simulink model "windpmsg11088"  (R2022b)
settings: Solver=VariableStepAuto  StartTime=0.0  StopTime=10  RelTol=1e-3
undefined symbols (not defined in the file or in its folder): sigbuilder_block
libraries: powerlib_extras x2, spsMeanLib x2, spsThreePhaseVIMeasurementLib x1, spsGroundLib x1, spsCurrentMeasurementLib x1, spsPermanentMagnetSynchronousMachineLib x1, spsThreePhaseSeriesRLCBranchLib x1, spsVoltageMeasurementLib x1, spspowerguiLib x1
settings Model: Creator=CC  LastModifiedBy=admin
settings SolverCC: AlgebraicLoopSolver=TrustRegion
settings DataIOCC: ReturnWorkspaceOutputs=off
settings DebuggingCC: UnconnectedInputMsg=warning  UnconnectedOutputMsg=warning  UnconnectedLineMsg=warning  SFMachineParentedDataDiag=warning  ArithmeticOperatorsInVariantConditions=warning
settings ModelReferenceCC: EnableRefExpFcnMdlSchedulingChecks=on
settings SFSimCC: SimUseLocalCustomCode=off  CustomCodeUndefinedFunction=UseInterfaceOnly
settings RTWCC: RTWUseLocalCustomCode=off

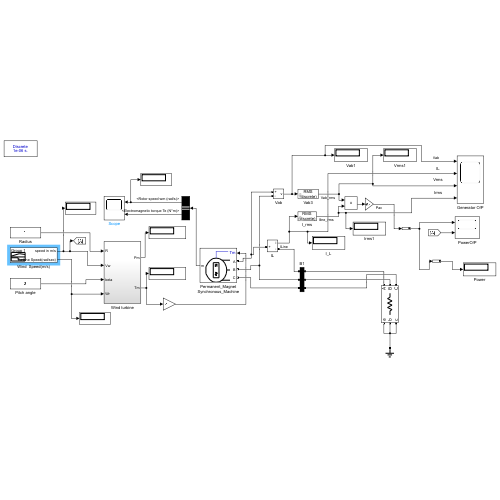
[thumbnail: Simulink's stored preview of the top-level diagram]
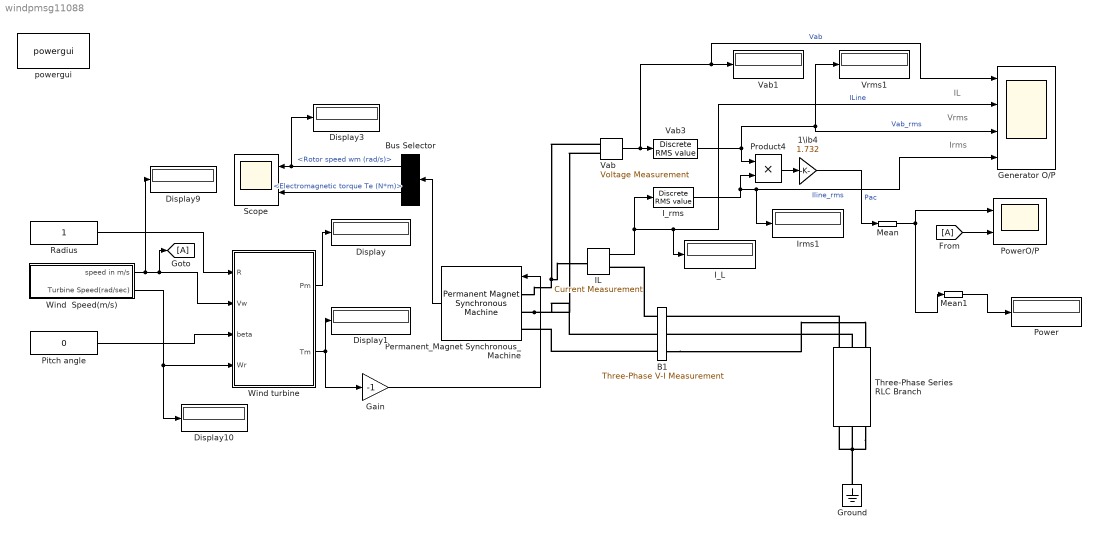
== system windpmsg11088 ==
  note: Irms
  note: Vrms
  note: IL
  1\ib4 : Gain  Gain=1.732  SaturateOnIntegerOverflow=on  OutDataTypeStr=Inherit: Same as input  ParamDataTypeStr=Inherit: Same as input
  B1 : spsThreePhaseVIMeasurementLib/Three-Phase V-I Measurement  VoltageMeasurement=phase-to-ground  SetLabelV=on  LabelV=Vabc_B1  Vpu=off  VpuLL=off  CurrentMeasurement=yes  SetLabelI=on  LabelI=Iabc_B1  Ipu=off  Pbase=100e6  Vbase=500e3  OutputType=Magnitude  PhasorSimulation=off  PSBequivalent=0
  Bus Selector : BusSelector  OutputSignals=Rotor speed wm (rad/s),Electromagnetic torque Te (N*m)
  Display{,1,3,9..10} (5 alike) : Display
      Display10 settings: Decimation=2
      Display9 settings: Decimation=2
  From : From
  Gain : Gain  Gain=-1
  Generator O/P : Scope  NumInputPorts=4
  Goto : Goto
  Ground : spsGroundLib/Ground  LConnTagsString=a
  IL : spsCurrentMeasurementLib/Current Measurement  PhasorSimulation=off  OutputType=Complex  PSBequivalent=0
  I_L : Display
      settings: SampleTime=1e-3
  I_rms : powerlib_extras/Discrete Measurements/Discrete  RMS value  Freq=50  Mag_Init=0  Ts=20e-6
  Irms1 : Display
      settings: SampleTime=1e-3
  Mean : spsMeanLib/Mean  Freq=50  Vinit=0  Ts=0
  Mean1 : spsMeanLib/Mean  Freq=50  Vinit=0  Ts=0
  Permanent_Magnet Synchronous_Machine : spsPermanentMagnetSynchronousMachineLib/Permanent Magnet Synchronous Machine  NbPhases=3  FluxDistribution=Sinusoidal  RotorType=Round  MechanicalLoad=Torque Tm  PresetModel=No  ShowDetailedParameters=on  MeasurementBus=off  Resistance=0.0485  Inductance=8.5e-3  dqInductances=[8.5e-3,8.5e-3]  La=0.000395  MachineConstant=Flux linkage established by magnets (V.s)  Flux=0.433  VoltageCst=392.6876  TorqueCst=3.2475  Flat=120  Mechanical=[0.01197 0.001189 5]  PolePairs=4  InitialConditions=[0,0, 0,0]  InitialConditions5ph=[0 0 0 0 0 0]  RefAngle=90 degrees behind phase A axis (modified Park)  IterativeDiscreteModel=Trapezoidal non iterative  TsBlock=-1  TsPowergui=0
  Pitch angle : Constant  Value=0
  Power : Display
      settings: SampleTime=1e-3
  PowerO/P : Scope  NumInputPorts=2
  Product4 : Product  RndMeth=Zero
  Radius : Constant
  Scope : Scope  NumInputPorts=2
  Three-Phase Series RLC Branch : spsThreePhaseSeriesRLCBranchLib/Three-Phase Series RLC Branch  LConnTagsString=A|B|C  RConnTagsString=A|B|C  BranchType=R  Resistance=30  Inductance=1e-3  Capacitance=10e-6  Measurements=None
  Vab : spsVoltageMeasurementLib/Voltage Measurement  PhasorSimulation=off  OutputType=Complex  PSBequivalent=0
  Vab1 : Display
      settings: SampleTime=1e-3
  Vab3 : powerlib_extras/Discrete Measurements/Discrete  RMS value  Freq=50  Mag_Init=0  Ts=20e-6
  Vrms1 : Display
      settings: SampleTime=1e-3
  Wind  Speed(m/s) : Subsystem  Tag=STV Subsys  LoadFcn=sigbuilder_block('load',[330.6 139.8 550.8 400.2 ]);  StartFcn=sigbuilder_block('start');  StopFcn=sigbuilder_block('stop');  ClipboardFcn=sigbuilder_block('clipboard');  mask(Sigbuilder block){tuvar=[0:10]}
      mask help: Simulink:masks:SigbuilderBlock_MD
      mask init:
      | if ~strcmp(get_param(bdroot(gcbh),'SimulationStatus'),'stopped') tuvar = sigbuilder_block('maskInit'); end
      settings: CopyFcn=sigbuilder_block('copy');  DeleteFcn=sigbuilder_block('delete');  ModelCloseFcn=sigbuilder_block('modelClose');  PreSaveFcn=sigbuilder_block('preSave');  PauseFcn=sigbuilder_block('pause');  ContinueFcn=sigbuilder_block('continue');  NameChangeFcn=sigbuilder_block('namechange');  OpenFcn=sigbuilder_block('open',[330.6 139.8 550.8 400.2 ]);  CloseFcn=sigbuilder_block('close');
      mask Display: plot(0, 0, 100, 100,[2, 2, 32, 32, 2], [68, 8, 8, 68, 68],[32, 2], [38, 38], [32, 19, 2],[53, 60, 44], [32, 17, 17, 2],[16, 16, 31, 31]);txt = getActiveGroup(gcbh);text(2, 100, txt,'verticalAlignment', 'top');
  Wind turbine : Subsystem
  powergui : spspowerguiLib/powergui  Priority=1  SimulationMode=Discrete  SampleTime=1e-6  frequency=60  Iterations=50  frequencyindice=0  Pbase=100e6  ErrMax=1e-4  UnitsV=kV  UnitsW=MW  buscounter=0  FunctionMessages=off  echomessages=off  EnableUseOfTLC=off  CurrentSourceSwitches=off  DisableSnubberDevices=off  DisableRonSwitches=off  DisableVfSwitches=off  DisplayEquations=off  AutomaticDiscreteSolvers=off  SolverType=Tustin/Backward Euler (TBE)  Interpol=off  ExternalGateDelay=off  methode=off  Ts=100  x0status=blocks  SPID=on  SwTol=0  HookPort=off  NonlinearTolerance=1e-4  nMaxIteration=100  ContinueOnMaxIteration=off  RestoreLinks=warning  ResistiveCurrentMeasurement=off  Frange=[0:2:500]  Ylog=off  Xlog=on  ShowGrid=off  save=off  variable=ZData  structure=0  ZoomFFT=off  StartTime=0.0  cycles=1  DisplayStyle=1  fundamental=60  FreqAxis=off  MaxFrequency=1000  frequencyindicesteady=1  RmsSteady=1  display=off
  wires:
  I_rms/1 -> Product4/2, Irms1/1, Generator O/P/4  "Iline_rms"
  Gain/1 -> Permanent_Magnet Synchronous_Machine/1
  Wind turbine/2(Tm) -> Gain/1, Display1/1
  IL/1 -> I_L/1, Generator O/P/2, I_rms/1  "ILine"
  Radius/1 -> Wind turbine/1(R)
  Vab/1 -> Vab1/1, Generator O/P/1, Vab3/1  "Vab"
  1\ib4/1 -> Mean/1  "Pac"
  Wind  Speed(m/s)/1(speed in m/s) -> Display9/1, Goto/1, Wind turbine/2(Vw)
  Product4/1 -> 1\ib4/1
  Wind turbine/1(Pm) -> Display/1
  Bus Selector/1 -> Display3/1, Scope/1  "<Rotor speed wm (rad/s)>"
  Bus Selector/2 -> Scope/2  "<Electromagnetic torque Te (N*m)>"
  Pitch angle/1 -> Wind turbine/3(beta)
  Vab3/1 -> Vrms1/1, Generator O/P/3, Product4/1  "Vab_rms"
  Permanent_Magnet Synchronous_Machine/1 -> Bus Selector/1
  Mean/1 -> Mean1/1, PowerO/P/1
  Wind  Speed(m/s)/2(Turbine Speed(rad/sec)) -> Display10/1, Wind turbine/4(Wr)
  From/1 -> PowerO/P/2
  Mean1/1 -> Power/1
  connections:
  Permanent_Magnet Synchronous_Machine/LConn1 -- IL/LConn1 -- Vab/LConn1
  Permanent_Magnet Synchronous_Machine/LConn2 -- B1/LConn2 -- Vab/LConn2
  Three-Phase Series RLC Branch/RConn3 -- Three-Phase Series RLC Branch/RConn1 -- Ground/LConn1 -- Three-Phase Series RLC Branch/RConn2
  B1/RConn3 -- Three-Phase Series RLC Branch/LConn3
  Three-Phase Series RLC Branch/LConn2 -- B1/RConn2
  Three-Phase Series RLC Branch/LConn1 -- B1/RConn1
  B1/LConn1 -- IL/RConn1
  B1/LConn3 -- Permanent_Magnet Synchronous_Machine/LConn3

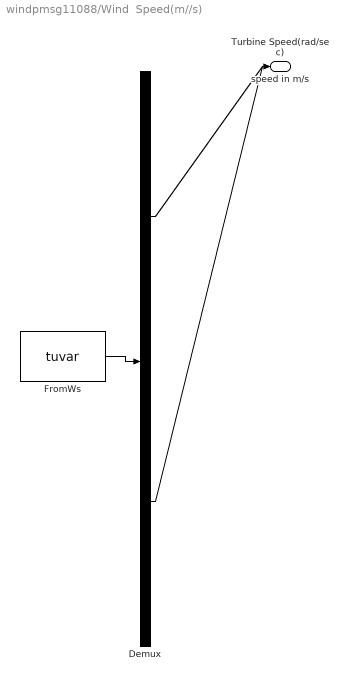
== system windpmsg11088/Wind  Speed(m//s) ==
  Demux : Demux  Tag=STV Demux  Outputs=2
      settings: DisplayOption=none
  FromWs : FromWorkspace  Tag=STV FromWs  VariableName=tuvar
      SigBuilderData=|
      | common.afterFinalStr = 'Extrapolate'
      | common.sampleTime = 0
      | dataSet.timeRange = [0 10]
      | dataSet.name = 'Group 1'
      | sbobj.Groups.Name = 'Group 1'
      | sbobj.Groups.Signals(1).Name = 'speed in m/s'
      | sbobj.Groups.Signals(1).XData = [0 1 2 3 4 5 6 7 8 9 10]
      | sbobj.Groups.Signals(1).YData = [10 10 10.4 12.4 11 12.4 9.2 9.6 13 11.6 13.3]
      | sbobj.Groups.Signals(2).Name = 'Turbine Speed(rad/sec)'
      | sbobj.Groups.Signals(2).XData = [0 1 2 3 4 5 6 7 8 9 10]
      | sbobj.Groups.Signals(2).YData = [66.9034 66.9034 69.5795 82.9602 73.5937 82.9602 61.5511 64.2273 86.9744 77.6079 88.9815]
  speed in m/s : Outport  Tag=STV Outport  VectorParamsAs1DForOutWhenUnconnected=off
  Turbine Speed(rad/sec) : Outport  Tag=STV Outport  Port=2  VectorParamsAs1DForOutWhenUnconnected=off
  wires:
  FromWs/1 -> Demux/1
  Demux/1 -> speed in m/s/1
  Demux/2 -> Turbine Speed(rad/sec)/1

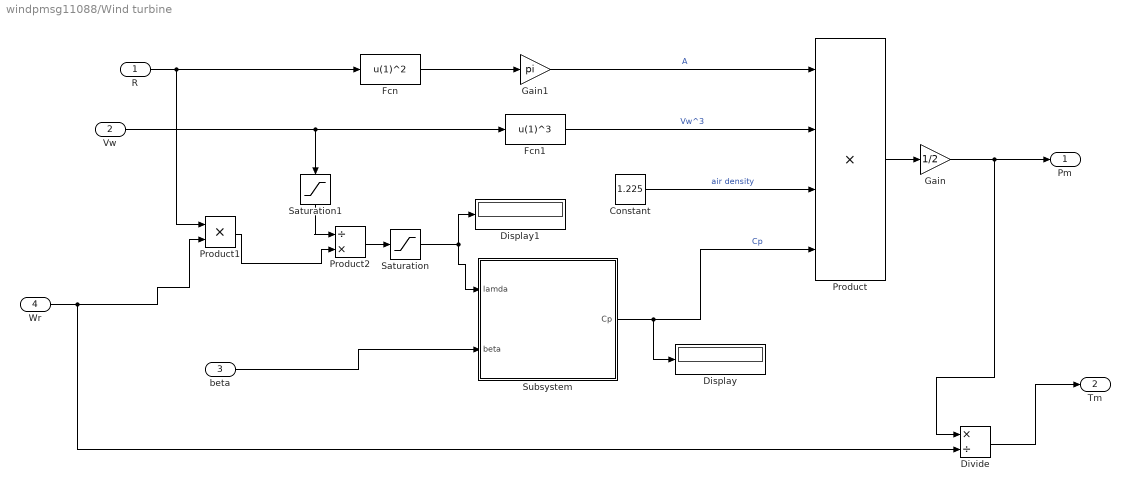
== system windpmsg11088/Wind turbine ==
  R : Inport
  Vw : Inport  Port=2
  beta : Inport  Port=3
  Wr : Inport  Port=4
  Constant : Constant  Value=1.225
  Display : Display
  Display1 : Display
  Divide : Product  Inputs=*/
  Fcn : Fcn  Expr=u(1)^2
  Fcn1 : Fcn  Expr=u(1)^3
  Gain : Gain  Gain=1/2
  Gain1 : Gain  Gain=pi
  Product : Product  Inputs=4
  Product1 : Product
  Product2 : Product  Inputs=/*
  Saturation : Saturate  UpperLimit=inf  LowerLimit=1e-6
  Saturation1 : Saturate  UpperLimit=inf  LowerLimit=1e-6
  Subsystem : Subsystem
  Pm : Outport  VectorParamsAs1DForOutWhenUnconnected=off
  Tm : Outport  Port=2  VectorParamsAs1DForOutWhenUnconnected=off
  wires:
  Gain1/1 -> Product/1  "A"
  Fcn1/1 -> Product/2  "Vw^3"
  Constant/1 -> Product/3  "air density"
  Subsystem/1(Cp) -> Display/1, Product/4  "Cp"
  Gain/1 -> Divide/1, Pm/1
  Product/1 -> Gain/1
  Fcn/1 -> Gain1/1
  R/1 -> Fcn/1, Product1/1
  Vw/1 -> Fcn1/1, Saturation1/1
  beta/1 -> Subsystem/2(beta)
  Wr/1 -> Divide/2, Product1/2
  Product1/1 -> Product2/2
  Product2/1 -> Saturation/1
  Saturation/1 -> Subsystem/1(lamda), Display1/1
  Saturation1/1 -> Product2/1
  Divide/1 -> Tm/1

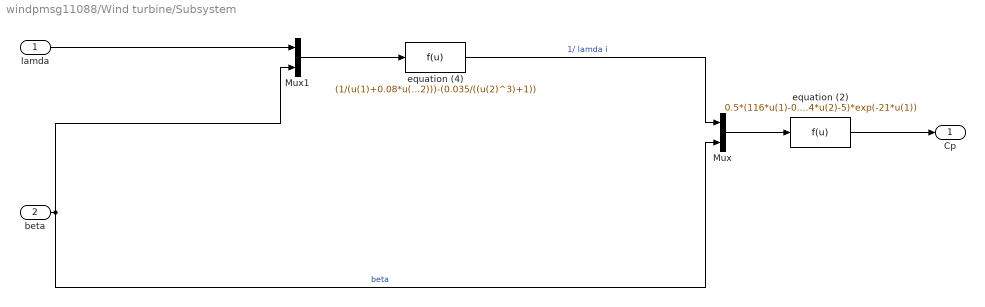
== system windpmsg11088/Wind turbine/Subsystem ==
  lamda : Inport
  beta : Inport  Port=2
  Mux : Mux  Inputs=2
  Mux1 : Mux  Inputs=2
  equation (2) : Fcn  Expr=0.5*(116*u(1)-0.4*u(2)-5)*exp(-21*u(1))
  equation (4) : Fcn  Expr=(1/(u(1)+0.08*u(2)))-(0.035/((u(2)^3)+1))
  Cp : Outport  VectorParamsAs1DForOutWhenUnconnected=off
  wires:
  equation (2)/1 -> Cp/1
  Mux/1 -> equation (2)/1
  equation (4)/1 -> Mux/1  "1/ lamda i"
  beta/1 -> Mux/2, Mux1/2  "beta"
  Mux1/1 -> equation (4)/1
  lamda/1 -> Mux1/1
